simulink model "SensingSubsystem_revA"  (R2021b)
settings: Solver=VariableStepAuto  StartTime=0.0  StopTime=stop_time  RelTol=1e-3
undefined symbols (not defined in the file or in its folder): chirp_params, chirps_to_capture, frame_params, peak_detection_params, plot_params, spectogram_params, waveform_params
libraries: simulink x3, hdlsllib x3, dspindex x3, dspsigops x2, radarlib x1, dspxfrm3 x1, phasedwavlib x1, dspswit3 x1
settings Model: Creator=David  LastModifiedBy=David

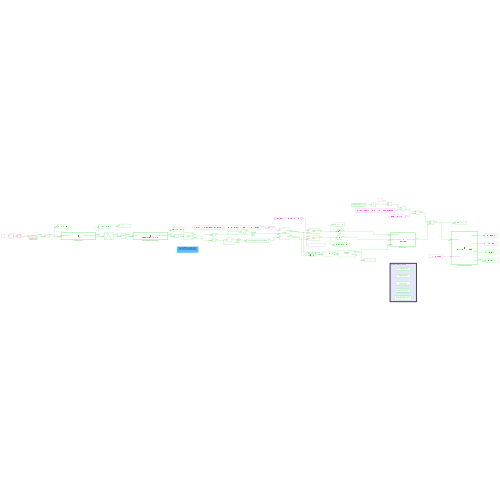
[thumbnail: Simulink's stored preview of the top-level diagram]
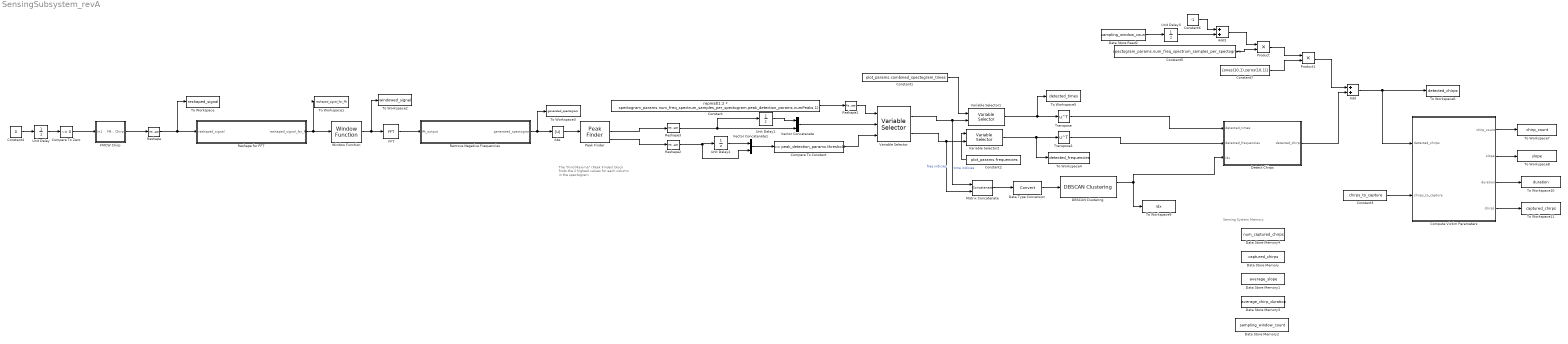
== system SensingSubsystem_revA ==
  note: Sensing System Memory
  note: The "Find Maxima" (Peak Finder)
      | block finds the 2 highest values
      | for each column in the spectogram
  Abs : Abs
  Add : Sum
  Add1 : Sum
  Compare To Constant : simulink/Logic and Bit Operations/Compare To Constant  relop=>=  const=peak_detection_params.threshold  OutDataTypeStr=boolean
  Compare To Zero : simulink/Logic and Bit Operations/Compare To Zero  relop=~=  OutDataTypeStr=boolean
  Compute Victim Parameters : MATLAB Function  TreatAsAtomicUnit=on
  Constant : Constant  Value=repmat(1:2 * spectogram_params.num_freq_spectrum_samples_per_spectogram,peak_detection_params.numPeaks,1)  VectorParams1D=off  OutDataTypeStr=uint32
  Constant1 : Constant  Value=plot_params.combined_spectogram_times
  Constant2 : Constant  Value=plot_params.frequencies
  Constant3 : Constant  Value=chirps_to_capture
  Constant4 : Constant  Value=0
  Constant5 : Constant  Value=spectogram_params.num_freq_spectrum_samples_per_spectogram
  Constant6 : Constant  Value=-1
  Constant7 : Constant  Value=[ones(10,1),zeros(10,1)]
  DBSCAN Clustering : radarlib/DBSCAN Clustering  BlockOutputs=Index and Cluster ID  EpsilonSource=Property  Epsilon=5  MinNumPoints=2  MaxNumPoints=10  EpsilonHistoryLength=10  EnableDisambiguation=off  AmbiguousDimension=1  SimulateUsing=Interpreted execution
      settings: SourceProductBaseCode=RA
  Data Store Memory : DataStoreMemory  DataStoreName=captured_chirps  ReadBeforeWriteMsg=warning  WriteAfterWriteMsg=warning  WriteAfterReadMsg=warning  InitialValue=zeros(chirps_to_capture, 2)  ShowAdditionalParam=off  OutDataTypeStr=double
  Data Store Memory1 : DataStoreMemory  DataStoreName=average_slope  ReadBeforeWriteMsg=warning  WriteAfterWriteMsg=warning  WriteAfterReadMsg=warning  ShowAdditionalParam=off  OutDataTypeStr=double
  Data Store Memory2 : DataStoreMemory  DataStoreName=sampling_window_count  ReadBeforeWriteMsg=warning  WriteAfterWriteMsg=warning  WriteAfterReadMsg=warning  InitialValue=-1  VectorParams1D=off  ShowAdditionalParam=off  OutDataTypeStr=int16
  Data Store Memory3 : DataStoreMemory  DataStoreName=average_chirp_duration  ReadBeforeWriteMsg=warning  WriteAfterWriteMsg=warning  WriteAfterReadMsg=warning  InitialValue=20  ShowAdditionalParam=off  OutDataTypeStr=double
  Data Store Memory4 : DataStoreMemory  DataStoreName=num_captured_chirps  ReadBeforeWriteMsg=warning  WriteAfterWriteMsg=warning  WriteAfterReadMsg=warning  ShowAdditionalParam=off  OutDataTypeStr=int16
  Data Store Read2 : DataStoreRead  DataStoreName=sampling_window_count  IndexOptions=Index vector (dialog)  Indices=1  OutputSizes=1
  Data Type Conversion : DataTypeConversion
  Detect Chirps : MATLAB Function  TreatAsAtomicUnit=on
  FFT : dspxfrm3/FFT  FFTImplementation=Auto  CompMethod=Table lookup  TableOpt=NEW  TableOptActive=Speed  BitRevOrder=off  Normalize=off  InheritFFTLength=on  FFTLength=64  WrapInput=on  roundingMode=Floor  overflowMode=off  firstCoeffDataTypeStr=Inherit: Same word length as input  firstCoeffLastDataTypeStr=Inherit: Same word length as input  outputMin=[]  outputMax=[]
  FMCW Chirp : Subsystem
  Matrix Concatenate : Concatenate  Mode=Multidimensional array  ConcatenateDimension=2
  Peak Finder : dspsigops/Peak Finder  polarity=Maxima  indexBase=One  outputIdx=on  outputVal=on  maxPeaks=peak_detection_params.numPeaks  NoiseDistinguish=off  thresh=1  roundingMode=Floor  overflowMode=off
      settings: SourceProductBaseCode=DS  allowOverrides=off
  Product : Product
  Product1 : Product
  Remove Negative Frequencies : MATLAB Function  TreatAsAtomicUnit=on
  Reshape : Reshape  OutputDimensionality=Customize  OutputDimensions=[50,50]
  Reshape for FFT : MATLAB Function  TreatAsAtomicUnit=on
  Reshape1 : Reshape
  Reshape2 : Reshape
  Reshape3 : Reshape
  To Workspace : ToWorkspace  VariableName=reshaped_signal  SampleTime=-1
      settings: MaxDataPoints=2
  To Workspace1 : ToWorkspace  VariableName=reshaped_signal_for_fft  SampleTime=-1
      settings: MaxDataPoints=2
  To Workspace10 : ToWorkspace  VariableName=duration  SampleTime=-1
      settings: MaxDataPoints=2
  To Workspace11 : ToWorkspace  VariableName=captured_chirps  SampleTime=-1
      settings: MaxDataPoints=2
  To Workspace2 : ToWorkspace  VariableName=windowed_signal  SampleTime=-1
      settings: MaxDataPoints=2
  To Workspace3 : ToWorkspace  VariableName=generated_spectogram  SampleTime=-1
      settings: MaxDataPoints=2
  To Workspace4 : ToWorkspace  VariableName=detected_frequencies  SampleTime=-1
      settings: MaxDataPoints=2
  To Workspace5 : ToWorkspace  VariableName=detected_times  SampleTime=-1
      settings: MaxDataPoints=2
  To Workspace6 : ToWorkspace  VariableName=detected_chirps  SampleTime=-1
      settings: MaxDataPoints=2
  To Workspace7 : ToWorkspace  VariableName=chirp_count  SampleTime=-1
      settings: MaxDataPoints=2
  To Workspace8 : ToWorkspace  VariableName=slope  SampleTime=-1
      settings: MaxDataPoints=2
  To Workspace9 : ToWorkspace  VariableName=idx  SampleTime=-1
      settings: MaxDataPoints=2
  Transpose : Math  Operator=transpose  SaturateOnIntegerOverflow=on
  Transpose1 : Math  Operator=transpose  SaturateOnIntegerOverflow=on
  Unit Delay : UnitDelay  InitialCondition=1  SampleTime=-1  HasFrameUpgradeWarning=on
  Unit Delay1 : UnitDelay  SampleTime=-1  HasFrameUpgradeWarning=on
  Unit Delay2 : UnitDelay  SampleTime=-1  HasFrameUpgradeWarning=on
  Unit Delay3 : UnitDelay  SampleTime=-1  HasFrameUpgradeWarning=on
  Variable Selector : dspindex/Variable Selector  NumInputs=2  rowsOrCols=Columns  IdxMode=Variable  Elements=[1 3]  ZerOneIdxMode=One-based  errmode=Clip Index  FillMode=on  FillValues=0
  Variable Selector1 : dspindex/Variable Selector  NumInputs=1  rowsOrCols=Rows  IdxMode=Variable  Elements=[1 3]  ZerOneIdxMode=One-based  errmode=Clip Index  FillMode=off  FillValues=0
  Variable Selector2 : dspindex/Variable Selector  NumInputs=1  rowsOrCols=Rows  IdxMode=Variable  Elements=[1 3]  ZerOneIdxMode=One-based  errmode=Clip Index  FillMode=off  FillValues=0
  Vector Concatenate : Concatenate
  Vector Concatenate1 : Concatenate
  Window Function : dspsigops/Window Function  winmode=Apply window to input  wintype=Hann  sampmode=Continuous  samptime=1  N=64  Rs=50  beta=10  winsamp=Symmetric  UserWindow=hamming  OptParams=off  UserParams={'symmetric'}  dataType=double  isSigned=on  wordLen=16  udDataType=sfix(16)  fracBitsMode=Best precision  numFracBits=15  roundingMode=Floor  overflowMode=off  numSidelobes=4  sidelobeLevel=-30
      settings: SourceProductBaseCode=DS
  wires:
  Reshape/1 -> Reshape for FFT/1(reshaped_signal), To Workspace/1
  FMCW Chirp/1(FMCW Chirp) -> Reshape/1
  Reshape for FFT/1(reshaped_signal_for_fft) -> Window Function/1, To Workspace1/1
  Window Function/1 -> FFT/1, To Workspace2/1
  FFT/1 -> Remove Negative Frequencies/1(fft_output)
  Remove Negative Frequencies/1(generated_spectogram) -> Abs/1, To Workspace3/1
  Abs/1 -> Peak Finder/1
  Constant/1 -> Reshape1/1
  Reshape1/1 -> Variable Selector/1
  Constant1/1 -> Variable Selector1/1
  Constant2/1 -> Variable Selector2/1
  Variable Selector/2 -> Matrix Concatenate/2, Variable Selector2/2  "freq indicies"
  Variable Selector2/1 -> To Workspace4/1, Transpose1/1
  Variable Selector1/1 -> To Workspace5/1, Transpose/1
  Detect Chirps/1(detected_chirps) -> Add/2
  Transpose/1 -> Detect Chirps/1(detected_times)
  Unit Delay/1 -> Compare To Zero/1
  Compare To Zero/1 -> FMCW Chirp/1(In1)
  Constant4/1 -> Unit Delay/1
  Transpose1/1 -> Detect Chirps/2(detected_frequencies)
  Variable Selector/1 -> Matrix Concatenate/1, Variable Selector1/2  "time indicies"
  Peak Finder/2 -> Reshape3/1
  Peak Finder/3 -> Reshape2/1
  Vector Concatenate1/1 -> Compare To Constant/1
  DBSCAN Clustering/1 -> Detect Chirps/3(idx), To Workspace9/1
  Matrix Concatenate/1 -> Data Type Conversion/1
  Data Type Conversion/1 -> DBSCAN Clustering/1
  Unit Delay1/1 -> Vector Concatenate/1
  Unit Delay2/1 -> Vector Concatenate1/1
  Reshape3/1 -> Vector Concatenate/2, Unit Delay1/1
  Vector Concatenate/1 -> Variable Selector/2
  Reshape2/1 -> Vector Concatenate1/2, Unit Delay2/1
  Compare To Constant/1 -> Variable Selector/3
  Constant5/1 -> Product/2
  Constant6/1 -> Add1/1
  Add1/1 -> Product/1
  Product/1 -> Product1/1
  Product1/1 -> Add/1
  Add/1 -> Compute Victim Parameters/1(detected_chirps), To Workspace6/1
  Constant7/1 -> Product1/2
  Unit Delay3/1 -> Add1/2
  Data Store Read2/1 -> Unit Delay3/1
  Compute Victim Parameters/1(chirp_count) -> To Workspace7/1
  Compute Victim Parameters/2(slope) -> To Workspace8/1
  Compute Victim Parameters/3(duration) -> To Workspace10/1
  Constant3/1 -> Compute Victim Parameters/2(chirps_to_capture)
  Compute Victim Parameters/4(chirps) -> To Workspace11/1

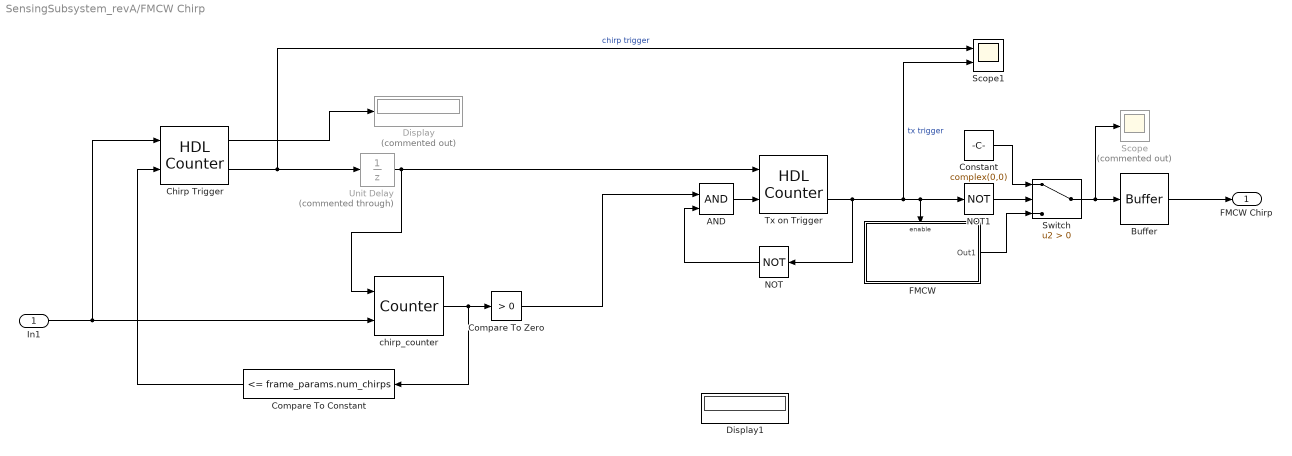
== system SensingSubsystem_revA/FMCW Chirp ==
  In1 : Inport
  AND : Logic  IconShape=distinctive  AllPortsSameDT=off  OutDataTypeStr=boolean
  Buffer : Buffer  N=int16(spectogram_params.num_ADC_samples_per_spectogram)  OutputFrames=off
  Chirp Trigger : hdlsllib/Sources/HDL Counter  CountType=Count limited  CountInit=1  CountStep=1  CountMax=waveform_params.sample_rate_Hz * waveform_params.sweep_time_s + chirp_params.num_samples_idle_time  CountFromType=Initial value  CountFrom=1  CountResetPort=on  CountLoadPort=off  CountEnbPort=on  CountDirPort=off  CountHitOutputPort=on  CountDataType=Unsigned  CountWordLen=16  CountFracLen=0  CountSampTime=1
  Compare To Constant : simulink/Logic and Bit Operations/Compare To Constant  relop=<=  const=frame_params.num_chirps  OutDataTypeStr=boolean
  Compare To Zero : hdlsllib/Logic and Bit Operations/Compare To Zero  relop=>  OutDataTypeStr=boolean
      settings: SourceProductBaseCode=SL
  Constant : Constant  Value=complex(0,0)
  Display : Display  Commented=on
  Display1 : Display
  FMCW : Subsystem
  NOT : Logic  Operator=NOT  IconShape=distinctive  AllPortsSameDT=off  OutDataTypeStr=boolean
  NOT1 : Logic  Operator=NOT  IconShape=distinctive  AllPortsSameDT=off  OutDataTypeStr=boolean
  Scope : Scope  Commented=on
  Scope1 : Scope  NumInputPorts=2
  Switch : Switch  Criteria=u2 > Threshold
  Tx on Trigger : hdlsllib/Sources/HDL Counter  CountType=Count limited  CountInit=1  CountStep=1  CountMax=chirp_params.num_samples_idle_time  CountFromType=Initial value  CountFrom=1  CountResetPort=on  CountLoadPort=off  CountEnbPort=on  CountDirPort=off  CountHitOutputPort=on  CountDataType=Unsigned  CountWordLen=16  CountFracLen=0  CountSampTime=1
  Unit Delay : UnitDelay  Commented=through  SampleTime=-1  HasFrameUpgradeWarning=on
  chirp_counter : dspswit3/Counter  Direction=Up  CountEvent=Rising edge  CounterSize=User defined  MaxCount=frame_params.num_chirps + 1  InitialCount=1  Output=Count  HitValue=32  ResetInput=on  SamplesPerFrame=1  Ts=1  CntDtype=int16  HitDtype=Logical
  FMCW Chirp : Outport
  wires:
  Buffer/1 -> FMCW Chirp/1
  chirp_counter/1 -> Compare To Constant/1, Compare To Zero/1
  Tx on Trigger/2 -> NOT/1, Scope1/2, FMCW/Enable, NOT1/1  "tx trigger"
  AND/1 -> Tx on Trigger/2
  Switch/1 -> Scope/1, Buffer/1
  FMCW/1(Out1) -> Switch/3
  NOT1/1 -> Switch/2
  Constant/1 -> Switch/1
  Chirp Trigger/1 -> Display/1
  Unit Delay/1 -> chirp_counter/1, Tx on Trigger/1
  Chirp Trigger/2 -> Scope1/1, Unit Delay/1  "chirp trigger"
  In1/1 -> chirp_counter/2, Chirp Trigger/1
  Compare To Zero/1 -> AND/1
  NOT/1 -> AND/2
  Compare To Constant/1 -> Chirp Trigger/2

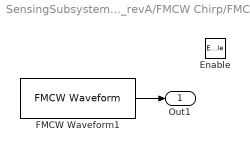
== system SensingSubsystem_revA/FMCW Chirp/FMCW ==
  Enable : EnablePort  StatesWhenEnabling=reset
  FMCW Waveform1 : phasedwavlib/FMCW Waveform  SampleRate=waveform_params.sample_rate_Hz  SweepTime=waveform_params.sweep_time_s  SweepBandwidth=waveform_params.sweep_BW_Hz  SweepDirection=Up  SweepInterval=Positive  OutputFormat=Samples  NumSamples=1  NumSweeps=waveform_params.num_sweeps  SimulateUsing=Interpreted execution
      settings: SourceProductBaseCode=AR
  Out1 : Outport
  wires:
  FMCW Waveform1/1 -> Out1/1

== matlab function SensingSubsystem_revA/Remove Negative Frequencies ==
  data: fft_output input; generated_spectogram output; half_fft_size parameter
function generated_spectogram = remove_negative_frequencies(fft_output, half_fft_size)
   
generated_spectogram = fft_output(1:half_fft_size,:);

== matlab function SensingSubsystem_revA/Reshape for FFT ==
  data: reshaped_signal input; reshaped_signal_for_fft output; fft_size parameter
function reshaped_signal_for_fft = reshape_for_fft(reshaped_signal, fft_size)
   
reshaped_signal_for_fft = reshaped_signal(1:fft_size,:);

== matlab function SensingSubsystem_revA/Detect Chirps ==
  data: detected_times input; detected_chirps output; detected_frequencies input; idx input; max_num_clusters parameter; sampling_window_count data_store_memory
function detected_chirps  = detect_chirps(detected_times,detected_frequencies,idx,max_num_clusters)
    %solve for the linear equation for each cluster provided there are enough
    %points
    threshold = 15;
    detected_chirps = zeros(max_num_clusters,2);
    global sampling_window_count;
    for cluster_id = 1:max(idx)
        %solve for linear model using linear algrebra
        %y is frequencies, x is time
        if sum(idx == cluster_id) > threshold && all(detected_times(idx == cluster_id))
            X = [ones(size(detected_times(idx == cluster_id),2),1),detected_times(idx == cluster_id).'];
            Y = detected_frequencies(idx == cluster_id).';
            B = inv(X.' * X) * X.' * Y;
            detected_chirps(cluster_id,1:2) = [-B(1)/B(2),B(2)];
        end
    end
    sampling_window_count = sampling_window_count + 1;
end

== matlab function SensingSubsystem_revA/Compute Victim Parameters ==
  data: detected_chirps input; average_chirp_duration data_store_memory; captured_chirps data_store_memory; average_slope data_store_memory; num_captured_chirps data_store_memory; chirp_count output; slope output; duration output; chirps_to_capture input; chirps output
function [chirp_count, slope, duration, chirps] = compute_victim_parameters(detected_chirps, chirps_to_capture)
    %declare global variables for accessing previously captured chirps, the
    %previously computed chirp duration, and the average slope
    global average_chirp_duration average_slope captured_chirps num_captured_chirps;
    for i = 1:size(detected_chirps,1)
        if detected_chirps(i,2) ~= 0 && num_captured_chirps < chirps_to_capture
            if num_captured_chirps == 0
                captured_chirps(1,:) = detected_chirps(i,:);
                num_captured_chirps = num_captured_chirps + 1;
            elseif all(abs(captured_chirps - detected_chirps(i,1)) > average_chirp_duration / 2,'all')
                captured_chirps(num_captured_chirps + 1,:) = detected_chirps(i,:);
                num_captured_chirps = num_captured_chirps + 1;
            end
            average_slope = sum(captured_chirps(1:num_captured_chirps,2))/ double(num_captured_chirps);
            if num_captured_chirps >= 2
                average_chirp_duration = (captured_chirps(num_captured_chirps,1) - captured_chirps(1,1))/double(num_captured_chirps - 1);
            end
            
        end
    end

    %output the new parameters for reference
    chirp_count = num_captured_chirps;
    slope = average_slope;
    duration = average_chirp_duration;
    chirps = captured_chirps;
end
